simulink model "TwoSwitch_Flyback_2024a"  (R2024a)
settings: Solver=ode45  StartTime=0.0  StopTime=10.0  MaxStep=SIM.Ts  RelTol=1e-3
undefined symbols (not defined in the file or in its folder): plecs, Ts
libraries: LossSim_Library x2
settings Model: Creator=Milan Utvic  LastModifiedBy=Tobias
settings SolverCC: InitialStep=SIM.Ts/2  AlgebraicLoopSolver=TrustRegion
settings DataIOCC: SaveFormat=StructureWithTime  ReturnWorkspaceOutputs=off
settings OptimizationCC: LifeSpan=inf
settings DebuggingCC: UnconnectedInputMsg=warning  UnconnectedOutputMsg=warning  UnconnectedLineMsg=warning  SFExecutionAtInitializationDiag=none  ArithmeticOperatorsInVariantConditions=warning
settings HardwareCC: ProdBitPerSizeT=32  ProdBitPerPtrDiffT=32  ProdWordSize=32  ProdHWDeviceType=Specified
settings ModelReferenceCC: EnableRefExpFcnMdlSchedulingChecks=on
settings SFSimCC: SimUseLocalCustomCode=off  CustomCodeUndefinedFunction=UseInterfaceOnly
settings RTWCC: RTWUseLocalCustomCode=off  GPUComputeCapability=3.5  DLArmComputeVersion=19.05
settings CodeAppCC: StateflowObjectComments=on

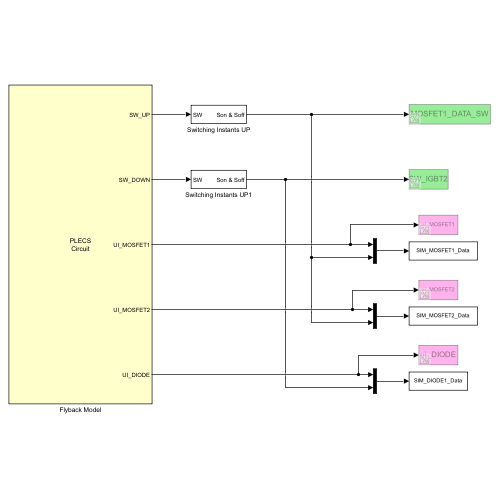
[thumbnail: Simulink's stored preview of the top-level diagram]
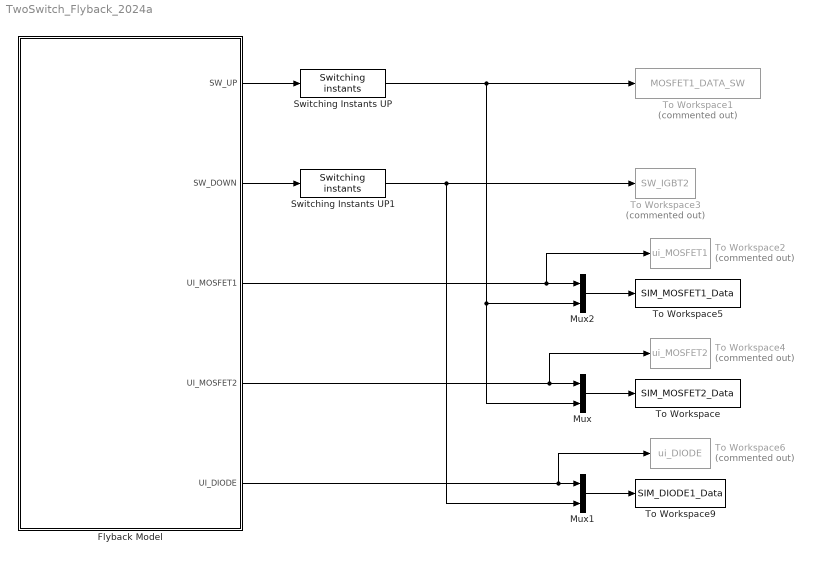
== system TwoSwitch_Flyback_2024a ==
  Flyback Model : Subsystem  LoadFcn=plecs('sl', 200);  InitFcn=plecs('sl', 214);  StartFcn=plecs('sl', 208);  StopFcn=plecs('sl', 209);  ClipboardFcn=plecs('sl', 212, 42);  mask(PlecsCircuit){PLECSData=<binary blob, 5200 chars, not shown>}
      mask prompts: PLECSData "PLECS Data (Do not delete or modify!)"
      mask init:
      | % PLACE CUSTOM INITIALIZATIONS ABOVE
      | % DO NOT REMOVE
      | plecs('sl', 215);
      | % DO NOT REMOVE
      settings: CopyFcn=plecs('sl', 203);  DeleteFcn=plecs('sl', 205);  UndoDeleteFcn=plecs('sl', 206);  PreSaveFcn=plecs('sl', 211);  PostSaveFcn=plecs('sl', 201);  NameChangeFcn=plecs('sl', 210);  DestroyFcn=plecs('sl', 207);  PreCopyFcn=plecs('sl', 216);  OpenFcn=plecs('sl', 202);  ErrorFcn=plerrorfcn
      mask Help: web(['file:///' fullfile(plecsdoc, 'creatingacircuit.html')])
      mask Display: disp('PLECS\nCircuit')
  Mux : Mux  Inputs=2
  Mux1 : Mux  Inputs=2
  Mux2 : Mux  Inputs=2
  Switching Instants UP : LossSim_Library/Switching instants  SystemSampleTime=-1  VariantActivationTime=update diagram  AllowFlexibleInterface=on  Latency=0  AutoFrameSizeCalculation=off
  Switching Instants UP1 : LossSim_Library/Switching instants  SystemSampleTime=-1  VariantActivationTime=update diagram  AllowFlexibleInterface=on  Latency=0  AutoFrameSizeCalculation=off
  To Workspace : ToWorkspace  VariableName=SIM_MOSFET2_Data  SampleTime=Ts
      settings: MaxDataPoints=NOS
  To Workspace1 : ToWorkspace  Commented=on  VariableName=MOSFET1_DATA_SW  SampleTime=Ts
      settings: MaxDataPoints=NOS
  To Workspace2 : ToWorkspace  Commented=on  VariableName=ui_MOSFET1  SampleTime=Ts
      settings: MaxDataPoints=NOS
  To Workspace3 : ToWorkspace  Commented=on  VariableName=SW_IGBT2  SampleTime=Ts
      settings: MaxDataPoints=NOS
  To Workspace4 : ToWorkspace  Commented=on  VariableName=ui_MOSFET2  SampleTime=Ts
      settings: MaxDataPoints=NOS
  To Workspace5 : ToWorkspace  VariableName=SIM_MOSFET1_Data  SampleTime=Ts
      settings: MaxDataPoints=NOS
  To Workspace6 : ToWorkspace  Commented=on  VariableName=ui_DIODE  SampleTime=Ts
      settings: MaxDataPoints=NOS
  To Workspace9 : ToWorkspace  VariableName=SIM_DIODE1_Data  SampleTime=Ts
      settings: MaxDataPoints=NOS
  wires:
  Switching Instants UP/1 -> To Workspace1/1, Mux2/2, Mux/2
  Mux/1 -> To Workspace/1
  Switching Instants UP1/1 -> To Workspace3/1, Mux1/2
  Mux1/1 -> To Workspace9/1
  Flyback Model/1(SW_UP) -> Switching Instants UP/1
  Flyback Model/2(SW_DOWN) -> Switching Instants UP1/1
  Flyback Model/3(UI_MOSFET1) -> To Workspace2/1, Mux2/1
  Flyback Model/5(UI_DIODE) -> To Workspace6/1, Mux1/1
  Mux2/1 -> To Workspace5/1
  Flyback Model/4(UI_MOSFET2) -> To Workspace4/1, Mux/1

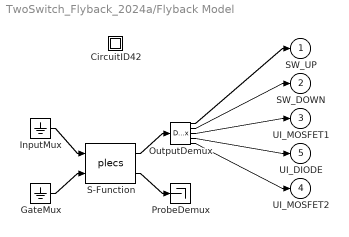
== system TwoSwitch_Flyback_2024a/Flyback Model ==
  " CircuitID42 " : Subsystem
  " GateMux " : Ground
  " InputMux " : Ground
  " OutputDemux " : Demux  Outputs=[ 1 1 2 2 2 ]
  " ProbeDemux " : Terminator
  " S-Function " : S-Function  FunctionName=plecs  SFunctionDeploymentMode=off  EnableBusSupport=off
  SW_UP : Outport  PortDimensions=1
  SW_DOWN : Outport  Port=2  PortDimensions=1
  UI_MOSFET1 : Outport  Port=3  PortDimensions=2
  UI_MOSFET2 : Outport  Port=4  PortDimensions=2
  UI_DIODE : Outport  Port=5  PortDimensions=2
  wires:
  " InputMux "/1 -> " S-Function "/1
  " GateMux "/1 -> " S-Function "/2
  " S-Function "/1 -> " OutputDemux "/1
  " S-Function "/2 -> " ProbeDemux "/1
  " OutputDemux "/1 -> SW_UP/1
  " OutputDemux "/2 -> SW_DOWN/1
  " OutputDemux "/3 -> UI_MOSFET1/1
  " OutputDemux "/4 -> UI_DIODE/1
  " OutputDemux "/5 -> UI_MOSFET2/1

== system TwoSwitch_Flyback_2024a/Flyback Model/ CircuitID42  ==
